simulink model "mcb_pmsm_foc_system"  (R2025b)
settings: Solver=FixedStepDiscrete  StartTime=0.0  StopTime=4  RelTol=1e-3  EnableMultiTasking=on
InitFcn:
  | mcb_pmsm_foc_qep_f28069LaunchPad_data;
  | mcb_algorithm_workflow_data;
values from neighbouring files (symbols this model uses):
  inverter = struct()    [mcb_pmsm_foc_qep_f28069LaunchPad_data.m]
  PI_params = mcb.getPIControllerParameters(pmsm, inverter, PU_System, T_pwm, Ts, Ts_speed)    [mcb_pmsm_foc_qep_f28069LaunchPad_data.m]
  pmsm = struct()    [mcb_pmsm_foc_qep_f28069LaunchPad_data.m]
  target = mcb.getProcessorParameters('F28069M', PWM_frequency)    [mcb_pmsm_foc_qep_f28069LaunchPad_data.m]
  Ts_motor = T_pwm/2    (= 1.66666666667e-05)    [mcb_pmsm_foc_qep_f28069LaunchPad_data.m]
  Ts_simulink = T_pwm/2    (= 1.66666666667e-05)    [mcb_pmsm_foc_qep_f28069LaunchPad_data.m]
undefined symbols (not defined in the file or in its folder): bit, Down, Enable, GPTRIP1SEL, GPTRIP2SEL, SpeedRef, TZ1, TZ2, Up
libraries: c2802xlib x5, c280xlib x5, c2806xlib x3, svdschedulerlib x1, simulink x1, mcbplantlib x1, mcbcontrolslib x1, autolibpmsmexterior x1
(part 2 of 2)

== system mcb_pmsm_foc_system/Embedded Processor/Hardware Init/Variant Subsystem/Code Generation/Calculate ADC Offset /If Action Subsystem3 ==
  Action Port : ActionPort
  Constant1 : Constant  Value=inverter.CtSensBOffset  OutDataTypeStr=Inherit: Inherit via back propagation
  Data Store Write2 : DataStoreWrite  DataStoreName=IbOffset  IndexOptions=Index vector (dialog)  Indices=1  OutputSizes=1
  wires:
  Constant1/1 -> Data Store Write2/1

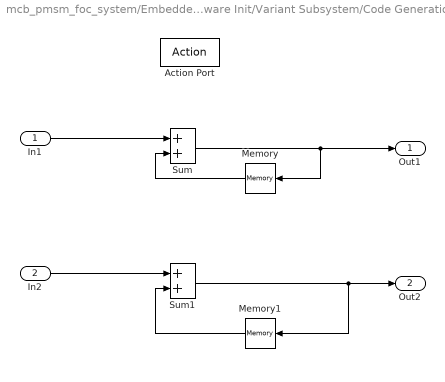
== system mcb_pmsm_foc_system/Embedded Processor/Hardware Init/Variant Subsystem/Code Generation/Calculate ADC Offset /For Iterator Subsystem/If Action Subsystem ==
  In1 : Inport
  In2 : Inport  Port=2
  Action Port : ActionPort
  Memory : Memory  InheritSampleTime=on
  Memory1 : Memory  InheritSampleTime=on
  Sum : Sum
  Sum1 : Sum
  Out1 : Outport
  Out2 : Outport  Port=2
  wires:
  In1/1 -> Sum/1
  Sum/1 -> Out1/1, Memory/1
  In2/1 -> Sum1/1
  Memory/1 -> Sum/2
  Sum1/1 -> Out2/1, Memory1/1
  Memory1/1 -> Sum1/2
